simulink model "n1_bernulli"  (Simulink 7.9)
settings: Solver=ode45  StartTime=0.0  StopTime=10000  RelTol=1e-3
libraries: simulink x1
settings Model: Creator=win7  LastModifiedBy=Антон

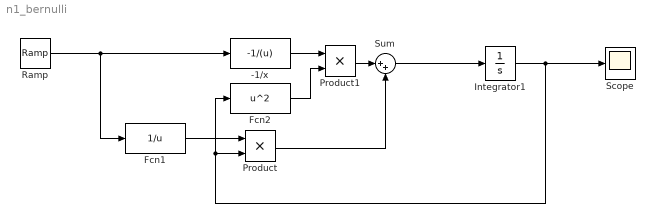
== system n1_bernulli ==
  -1/x : Fcn  Expr=-1/(u)
  Fcn1 : Fcn  Expr=1/u
  Fcn2 : Fcn  Expr=u^2
  Integrator1 : Integrator  InitialCondition=0.0001
  Product : Product  RndMeth=Zero
  Product1 : Product  RndMeth=Zero
  Ramp : simulink/Sources/Ramp  slope=1  start=1  X0=1
  Scope : Scope
      settings: TimeRange=35  YMin=-1  YMax=1
  Sum : Sum  Inputs=|++
  wires:
  Integrator1/1 -> Product/2, Fcn2/1, Scope/1
  Fcn1/1 -> Product/1
  Ramp/1 -> Fcn1/1, -1/x/1
  -1/x/1 -> Product1/1
  Fcn2/1 -> Product1/2
  Product1/1 -> Sum/1
  Product/1 -> Sum/2
  Sum/1 -> Integrator1/1
